simulink model "chap1_19"  (Simulink 6.3)
settings: Solver=ode45  StartTime=0.0  StopTime=1.0  RelTol=1e-3
values from neighbouring files (symbols this model uses):
  ki = 2.0    (= 2)    [chap1_10.m]    (also in chap1_12.m = 0.1; chap1_13.m = 0.005; chap1_14int.m = 0.05; chap1_15.m = 9)
  kp = 1.0    (= 1)    [chap1_10.m]    (also in chap1_12.m = 8; chap1_13.m = 0.8; chap1_14int.m = 1.8; chap1_15.m = 0.85)
  ts = 0.001    [chap1_10.m]    (also in chap1_12.m; chap1_13.m = 20; chap1_14int.m = 20; chap1_15.m)
undefined symbols (not defined in the file or in its folder): den, denQ, DiscIntNeverNeededParam, num, numQ
libraries: simulink x1
settings Model: LastModifiedBy=Administrator  ExtModeTrigMode=oneshot  ExtModeArmWhenConnect=off  StrictBusMsg=None
settings DataIOCC: LimitDataPoints=off
settings OptimizationCC: BlockReduction=off  BooleanDataType=off
settings DebuggingCC: SolverPrmCheckMsg=none
settings HardwareCC: TargetUnknown=on

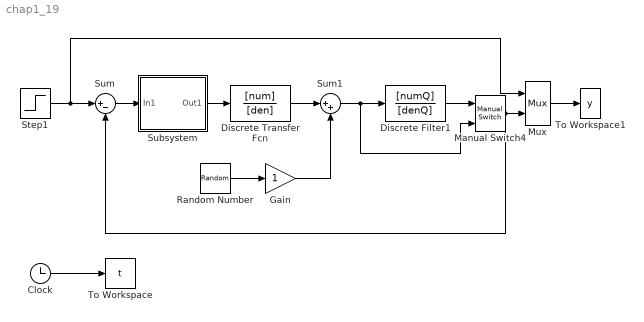
== system chap1_19 ==
  Clock : Clock
      settings: Decimation=10
  Discrete Transfer Fcn : DiscreteTransferFcn  Numerator=[num]  Denominator=[den]  SampleTime=ts
  Discrete Filter1 : DiscreteFilter  Numerator=[numQ]  Denominator=[denQ]  SampleTime=ts
  Gain : Gain  SaturateOnIntegerOverflow=on
  Manual Switch4 : simulink/Signal Routing/Manual Switch  sw=1  action=0
  Mux : Mux  Inputs=2
  Random Number : RandomNumber  SampleTime=ts
  Step1 : Step  Time=0  After=20  SampleTime=ts
  Subsystem : Subsystem
  Sum : Sum  Inputs=|+-  SaturateOnIntegerOverflow=on  InputSameDT=on
  Sum1 : Sum  Inputs=|++  SaturateOnIntegerOverflow=on  InputSameDT=on
  To Workspace : ToWorkspace  VariableName=t  SampleTime=-1  SaveFormat=Array
  To Workspace1 : ToWorkspace  VariableName=y  SampleTime=-1  SaveFormat=Array
  wires:
  Discrete Transfer Fcn/1 -> Sum1/1
  Discrete Filter1/1 -> Manual Switch4/1
  Sum1/1 -> Discrete Filter1/1, Manual Switch4/2
  Subsystem/1(Out1) -> Discrete Transfer Fcn/1
  Mux/1 -> To Workspace1/1
  Manual Switch4/1 -> Sum/2, Mux/2
  Step1/1 -> Sum/1, Mux/1
  Random Number/1 -> Gain/1
  Sum/1 -> Subsystem/1(In1)
  Gain/1 -> Sum1/2
  Clock/1 -> To Workspace/1

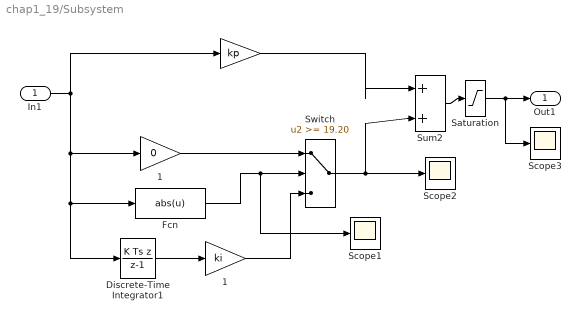
== system chap1_19/Subsystem ==
  In1 : Inport
  "  " : Gain  Gain=kp  SaturateOnIntegerOverflow=on
  "   1" : Gain  Gain=0  SaturateOnIntegerOverflow=on
  " 1" : Gain  Gain=ki  SaturateOnIntegerOverflow=on
  Discrete-Time Integrator1 : DiscreteIntegrator  IntegratorMethod=Integration: Backward Euler  SampleTime=ts  ICPrevOutput=DiscIntNeverNeededParam  ICPrevScaledInput=DiscIntNeverNeededParam
  Fcn : Fcn  Expr=abs(u)
  Saturation : Saturate  UpperLimit=10  LowerLimit=-10
  Scope1 : Scope
  Scope2 : Scope
  Scope3 : Scope
  Sum2 : Sum  Inputs=|++  SaturateOnIntegerOverflow=on  InputSameDT=on
  Switch : Switch  Threshold=19.20  SaturateOnIntegerOverflow=on  InputSameDT=on
  Out1 : Outport
  wires:
  "  "/1 -> Sum2/1
  Sum2/1 -> Saturation/1
  In1/1 -> "  "/1, "   1"/1, Discrete-Time Integrator1/1, Fcn/1
  Discrete-Time Integrator1/1 -> " 1"/1
  "   1"/1 -> Switch/1
  " 1"/1 -> Switch/3
  Fcn/1 -> Switch/2, Scope1/1
  Switch/1 -> Sum2/2, Scope2/1
  Saturation/1 -> Out1/1, Scope3/1
